simulink model "LookupTableDynamic2"  (R2014a)
settings: Solver=ode45  StartTime=0.0  StopTime=10.0  RelTol=1e-3
libraries: simulink x1
settings Model: CovSFcnEnable=on  BufferReuse=off  Creator=yamasefu  LastModifiedBy=ts1413
settings OptimizationCC: SimCompilerOptimization=off
settings DebuggingCC: MergeDetectMultiDrivingBlocksExec=error  SolverPrmCheckMsg=none  FrameProcessingCompatibilityMsg=error
settings RTWCC: RTWCompilerOptimization=off

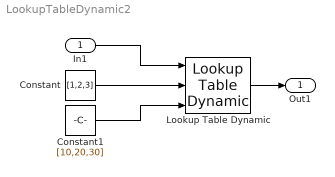
== system LookupTableDynamic2 ==
  In1 : Inport
  Constant : Constant  Value=[1,2,3]
  Constant1 : Constant  Value=[10,20,30]
  Lookup Table Dynamic : simulink/Lookup Tables/Lookup Table Dynamic  LookUpMeth=Interpolation-Extrapolation  OutDataTypeStr=fixdt('double')  OutputDataTypeScalingMode=Specify via dialog  OutDataType=fixdt('double')  OutScaling=2^-10  DoSatur=off
  Out1 : Outport
  wires:
  In1/1 -> Lookup Table Dynamic/1
  Constant/1 -> Lookup Table Dynamic/2
  Constant1/1 -> Lookup Table Dynamic/3
  Lookup Table Dynamic/1 -> Out1/1
